simulink model "pruebas_control_posicion"  (R2023b)
settings: Solver=VariableStepAuto  StartTime=0.0  StopTime=10  MaxStep=1e-5  RelTol=1e-3
values from neighbouring files (symbols this model uses):
  r = 120.0    (= 120)    [diagrama_polos_y_ceros_LTI.m]    (also in main.m; parametros.m)
settings Model: Creator=nicol  LastModifiedBy=nicol

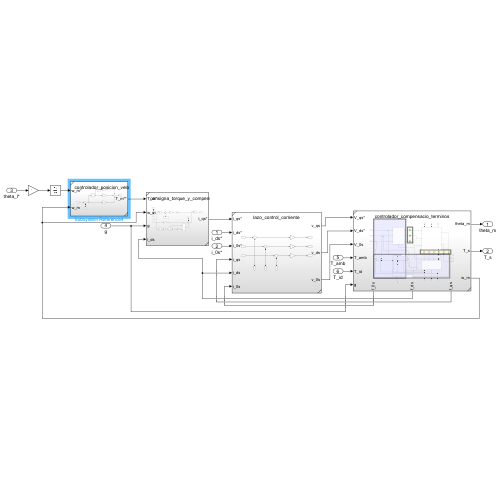
[thumbnail: Simulink's stored preview of the top-level diagram]
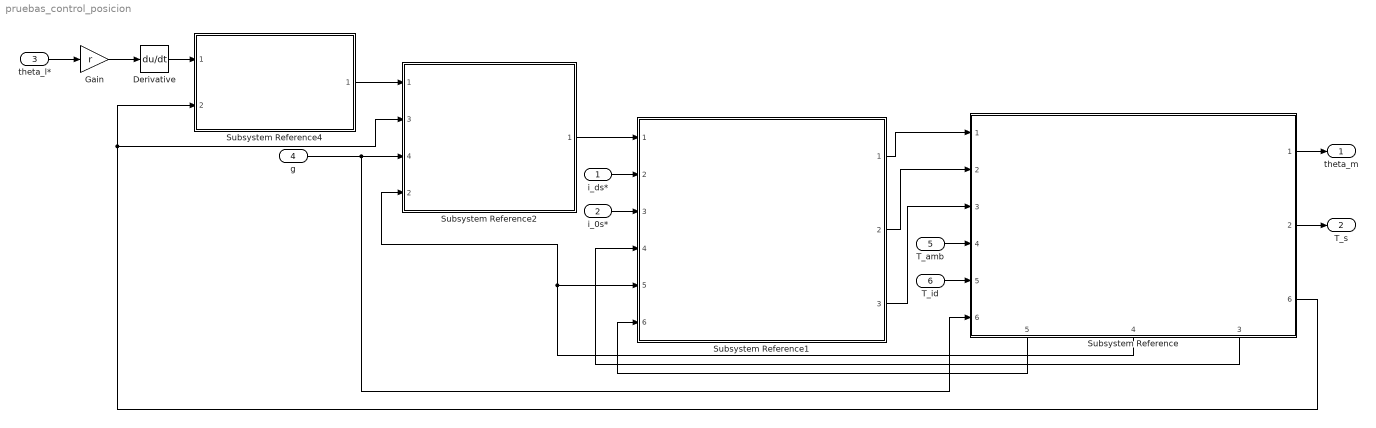
== system pruebas_control_posicion ==
  i_ds* : Inport
  i_0s* : Inport  Port=2
  theta_l* : Inport  Port=3
  g : Inport  Port=4
  T_amb : Inport  Port=5
  T_id : Inport  Port=6
  Derivative : Derivative
  Gain : Gain  Gain=r
  Subsystem Reference : Subsystem  ReferencedSubsystem=controlador_compensacio_terminos
      settings: PortSchema="{\"entries\":[{\"content\":{\"sides\":[{\"content\":{\"connectorIds\":[\"In1\",\"In2\",\"In3\",\"In4\",\"In5\",\"In6\"]},\"type\":\"ConnectorPlacement.EquallySpacedRectSide\",\"uuid\":\"b1c276fb-f5d1-4d19-a6ea-7d1a09b8349f\"},{\"content\":{\"connectorIds\":[\"Out1\",\"Out2\",\"Out6\"],\"side\":\"RIGHT\"},\"type\":\"ConnectorPlacement.EquallySpacedRectSide\",\"uuid\":\"27d8bc07-3c44-4620-a597-2ff8ea4c23ab\"},{\"content\":{\"side\":\"TOP\"},\"type\":\"ConnectorPlacement.EquallySpacedRectSide\",\"uuid\":\"3df4da6c-73e7-44ec-b643-950781e1e40a\"},{\"content\":{\"connectorIds\":[\"Out5\",\"Out4\",\"Out3\"],\"side\":\"BOTTOM\"},\"type\":\"ConnectorPlacement.EquallySpacedRectSide\",\"uuid\":\"41447b30-fc5c-45b8-8eff-edc74dd03fa8\"}]},\"type\":\"ConnectorPlacement.EquallySpacedConnector\",\"uuid\":\"40e819b3-95dd-49e4-ad1c-9b4691395cc7\"}],\"packageUris\":[\"http://schema.mathworks.com/mf0/Connector/R2020b\"],\"version\":\"1.0\"}"
  Subsystem Reference1 : Subsystem  ReferencedSubsystem=lazo_control_corriente
  Subsystem Reference2 : Subsystem  ReferencedSubsystem=consigna_torque_y_compensaciones
      settings: PortSchema="{\"entries\":[{\"content\":{\"sides\":[{\"content\":{\"connectorIds\":[\"In1\",\"In3\",\"In4\",\"In2\"]},\"type\":\"ConnectorPlacement.EquallySpacedRectSide\",\"uuid\":\"1885e5f5-f6ac-4449-9525-6488a0e1a0df\"},{\"content\":{\"connectorIds\":[\"Out1\"],\"side\":\"RIGHT\"},\"type\":\"ConnectorPlacement.EquallySpacedRectSide\",\"uuid\":\"5c837a64-ddee-40b5-814c-ed51094d23eb\"},{\"content\":{\"side\":\"TOP\"},\"type\":\"ConnectorPlacement.EquallySpacedRectSide\",\"uuid\":\"3b41ea9d-e5d3-43cd-ba13-1502040c9f0f\"}]},\"type\":\"ConnectorPlacement.EquallySpacedConnector\",\"uuid\":\"b9cdf7e5-86b7-4e3e-be26-3bae3f56036b\"}],\"packageUris\":[\"http://schema.mathworks.com/mf0/Connector/R2020b\"],\"version\":\"1.0\"}"
  Subsystem Reference4 : Subsystem  ReferencedSubsystem=controlador_posicion_velocidad
  theta_m : Outport
  T_s : Outport  Port=2
  wires:
  Subsystem Reference1/3 -> Subsystem Reference/3
  Subsystem Reference1/2 -> Subsystem Reference/2
  Subsystem Reference1/1 -> Subsystem Reference/1
  Subsystem Reference2/1 -> Subsystem Reference1/1
  Subsystem Reference4/1 -> Subsystem Reference2/1
  Subsystem Reference/5 -> Subsystem Reference1/6
  Subsystem Reference/4 -> Subsystem Reference1/5, Subsystem Reference2/2
  Subsystem Reference/3 -> Subsystem Reference1/4
  Derivative/1 -> Subsystem Reference4/1
  i_ds*/1 -> Subsystem Reference1/2
  i_0s*/1 -> Subsystem Reference1/3
  Subsystem Reference/6 -> Subsystem Reference4/2, Subsystem Reference2/3
  Gain/1 -> Derivative/1
  theta_l*/1 -> Gain/1
  g/1 -> Subsystem Reference/6, Subsystem Reference2/4
  T_amb/1 -> Subsystem Reference/4
  T_id/1 -> Subsystem Reference/5
  Subsystem Reference/1 -> theta_m/1
  Subsystem Reference/2 -> T_s/1
